simulink model "ConSys_A1"  (Simulink 8.3)
settings: Solver=ode3  StartTime=0.0  StopTime=Time(end)  FixedStep=Ts  RelTol=1e-3
values from neighbouring files (symbols this model uses):
  d = r*h    (= 1.6)    [StartUp_A1.m]
  d0 = d*h    (= 0.0032)    [StartUp_A1.m]
  h = 0.002    [StartUp_A1.m]
  Ka = diag([ 3  20  20  150  355  520])    [StartUp_A1.m]
  Kd = diag([ 3   5  25  100   15 1050])    [StartUp_A1.m]
  Ki = diag([35 555 810 7410 1850 5815])    [StartUp_A1.m]
  Kp = diag([55 180 350 1960  680 4450])    [StartUp_A1.m]
  r = 800    [StartUp_A1.m]
  TD = ss(Atd,Btd,Ctd,Dtd,Ts)    [StartUp_A1.m]
  Ts = 1/200    (= 0.005)    [StartUp_A1.m]
undefined symbols (not defined in the file or in its folder): DiscIntNeverNeededParam
undefined symbols (not defined in the file): ADAMS_cwd, ADAMS_exec, ADAMS_host, ADAMS_init, ADAMS_inputs, ADAMS_outputs, ADAMS_prefix, ADAMS_static, ADAMS_sysdir
libraries: cstblocks x6
(part 2 of 9)

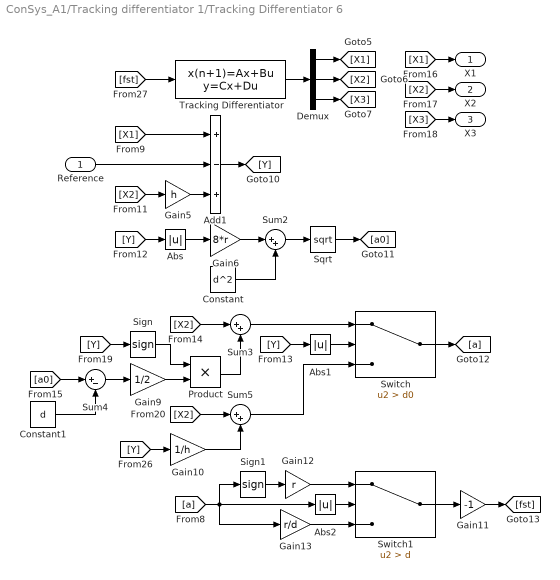
== system ConSys_A1/Tracking differentiator 1/Tracking Differentiator 6 ==
  Reference : Inport
  Abs : Abs
  Abs1 : Abs
  Abs2 : Abs
  Add1 : Sum  Inputs=+-+
  Constant : Constant  Value=d^2
  Constant1 : Constant  Value=d
  Demux : Demux  Outputs=3
  Gain10 : Gain  Gain=1/h
  Gain11 : Gain  Gain=-1
  Gain12 : Gain  Gain=r
  Gain13 : Gain  Gain=r/d
  Gain5 : Gain  Gain=h
  Gain6 : Gain  Gain=8*r
  Gain9 : Gain  Gain=1/2
  Product : Product
  Sign : Signum
  Sign1 : Signum
  Sqrt : Sqrt  SaturateOnIntegerOverflow=on
  Sum2 : Sum  Inputs=|++
  Sum3 : Sum  Inputs=|++
  Sum4 : Sum  Inputs=|+-
  Sum5 : Sum  Inputs=|++
  Switch : Switch  Criteria=u2 > Threshold  Threshold=d0
  Switch1 : Switch  Criteria=u2 > Threshold  Threshold=d
  Tracking Differentiator : DiscreteStateSpace  A=TD.a  B=TD.b  C=TD.c  D=TD.d  SampleTime=Ts
  X1 : Outport
  X2 : Outport  Port=2
  X3 : Outport  Port=3
  wires:
  Gain11/1 -> [fst]
  Abs2/1 -> Switch1/2
  [Y] -> Gain10/1
  Sum5/1 -> Switch/3
  Switch/1 -> [a]
  [Y] -> Sign/1
  Switch1/1 -> Gain11/1
  [a] -> Abs2/1, Sign1/1, Gain13/1
  Gain10/1 -> Sum5/2
  [fst] -> Tracking Differentiator/1
  [X2] -> Sum5/1
  Constant1/1 -> Sum4/2
  Sign/1 -> Product/1
  Product/1 -> Sum3/2
  [a0] -> Sum4/1
  Gain13/1 -> Switch1/3
  Sum4/1 -> Gain9/1
  [X2] -> Sum3/1
  Sum3/1 -> Switch/1
  [Y] -> Abs1/1
  Gain9/1 -> Product/2
  Sign1/1 -> Gain12/1
  Abs1/1 -> Switch/2
  Sum2/1 -> Sqrt/1
  Sqrt/1 -> [a0]
  Constant/1 -> Sum2/2
  Abs/1 -> Gain6/1
  Gain6/1 -> Sum2/1
  [Y] -> Abs/1
  Demux/2 -> [X2]
  Tracking Differentiator/1 -> Demux/1
  Demux/3 -> [X3]
  Demux/1 -> [X1]
  Add1/1 -> [Y]
  [X1] -> X1/1
  Reference/1 -> Add1/2
  [X2] -> Gain5/1
  [X2] -> X2/1
  Gain12/1 -> Switch1/1
  [X1] -> Add1/1
  Gain5/1 -> Add1/3
  [X3] -> X3/1

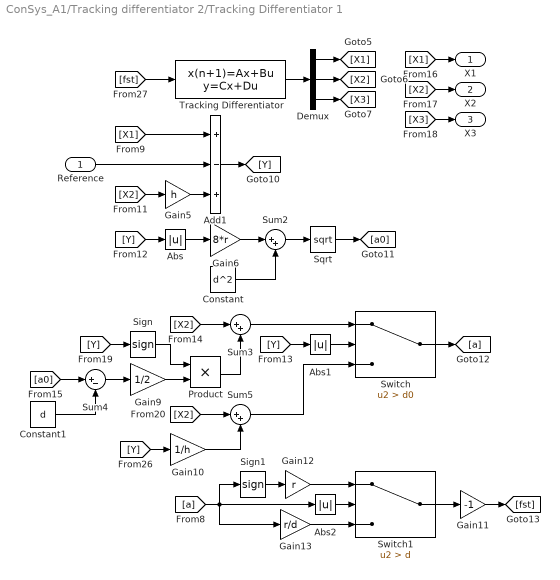
== system ConSys_A1/Tracking differentiator 2/Tracking Differentiator 1 ==
  Reference : Inport
  Abs : Abs
  Abs1 : Abs
  Abs2 : Abs
  Add1 : Sum  Inputs=+-+
  Constant : Constant  Value=d^2
  Constant1 : Constant  Value=d
  Demux : Demux  Outputs=3
  Gain10 : Gain  Gain=1/h
  Gain11 : Gain  Gain=-1
  Gain12 : Gain  Gain=r
  Gain13 : Gain  Gain=r/d
  Gain5 : Gain  Gain=h
  Gain6 : Gain  Gain=8*r
  Gain9 : Gain  Gain=1/2
  Product : Product
  Sign : Signum
  Sign1 : Signum
  Sqrt : Sqrt  SaturateOnIntegerOverflow=on
  Sum2 : Sum  Inputs=|++
  Sum3 : Sum  Inputs=|++
  Sum4 : Sum  Inputs=|+-
  Sum5 : Sum  Inputs=|++
  Switch : Switch  Criteria=u2 > Threshold  Threshold=d0
  Switch1 : Switch  Criteria=u2 > Threshold  Threshold=d
  Tracking Differentiator : DiscreteStateSpace  A=TD.a  B=TD.b  C=TD.c  D=TD.d  SampleTime=Ts
  X1 : Outport
  X2 : Outport  Port=2
  X3 : Outport  Port=3
  wires:
  Gain11/1 -> [fst]
  Abs2/1 -> Switch1/2
  [Y] -> Gain10/1
  Sum5/1 -> Switch/3
  Switch/1 -> [a]
  [Y] -> Sign/1
  Switch1/1 -> Gain11/1
  [a] -> Abs2/1, Sign1/1, Gain13/1
  Gain10/1 -> Sum5/2
  [fst] -> Tracking Differentiator/1
  [X2] -> Sum5/1
  Constant1/1 -> Sum4/2
  Sign/1 -> Product/1
  Product/1 -> Sum3/2
  [a0] -> Sum4/1
  Gain13/1 -> Switch1/3
  Sum4/1 -> Gain9/1
  [X2] -> Sum3/1
  Sum3/1 -> Switch/1
  [Y] -> Abs1/1
  Gain9/1 -> Product/2
  Sign1/1 -> Gain12/1
  Abs1/1 -> Switch/2
  Sum2/1 -> Sqrt/1
  Sqrt/1 -> [a0]
  Constant/1 -> Sum2/2
  Abs/1 -> Gain6/1
  Gain6/1 -> Sum2/1
  [Y] -> Abs/1
  Demux/2 -> [X2]
  Tracking Differentiator/1 -> Demux/1
  Demux/3 -> [X3]
  Demux/1 -> [X1]
  Add1/1 -> [Y]
  [X1] -> X1/1
  Reference/1 -> Add1/2
  [X2] -> Gain5/1
  [X2] -> X2/1
  Gain12/1 -> Switch1/1
  [X1] -> Add1/1
  Gain5/1 -> Add1/3
  [X3] -> X3/1

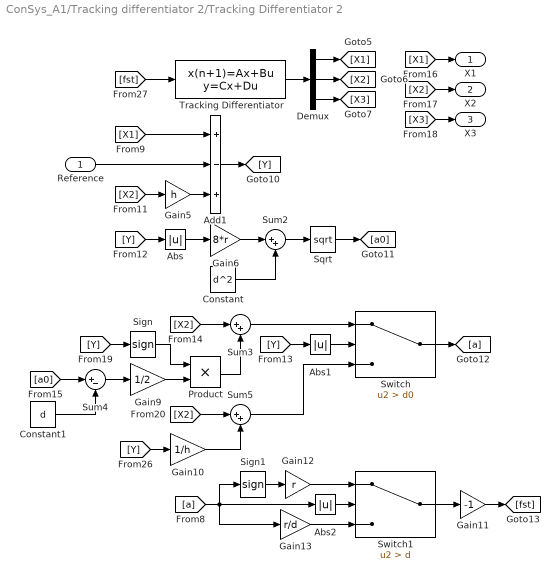
== system ConSys_A1/Tracking differentiator 2/Tracking Differentiator 2 ==
  Reference : Inport
  Abs : Abs
  Abs1 : Abs
  Abs2 : Abs
  Add1 : Sum  Inputs=+-+
  Constant : Constant  Value=d^2
  Constant1 : Constant  Value=d
  Demux : Demux  Outputs=3
  Gain10 : Gain  Gain=1/h
  Gain11 : Gain  Gain=-1
  Gain12 : Gain  Gain=r
  Gain13 : Gain  Gain=r/d
  Gain5 : Gain  Gain=h
  Gain6 : Gain  Gain=8*r
  Gain9 : Gain  Gain=1/2
  Product : Product
  Sign : Signum
  Sign1 : Signum
  Sqrt : Sqrt  SaturateOnIntegerOverflow=on
  Sum2 : Sum  Inputs=|++
  Sum3 : Sum  Inputs=|++
  Sum4 : Sum  Inputs=|+-
  Sum5 : Sum  Inputs=|++
  Switch : Switch  Criteria=u2 > Threshold  Threshold=d0
  Switch1 : Switch  Criteria=u2 > Threshold  Threshold=d
  Tracking Differentiator : DiscreteStateSpace  A=TD.a  B=TD.b  C=TD.c  D=TD.d  SampleTime=Ts
  X1 : Outport
  X2 : Outport  Port=2
  X3 : Outport  Port=3
  wires:
  [X3] -> X3/1
  Gain5/1 -> Add1/3
  [X1] -> Add1/1
  Gain12/1 -> Switch1/1
  [X2] -> X2/1
  [X2] -> Gain5/1
  Reference/1 -> Add1/2
  [X1] -> X1/1
  Add1/1 -> [Y]
  Demux/1 -> [X1]
  Demux/3 -> [X3]
  Tracking Differentiator/1 -> Demux/1
  Demux/2 -> [X2]
  [Y] -> Abs/1
  Gain6/1 -> Sum2/1
  Abs/1 -> Gain6/1
  Constant/1 -> Sum2/2
  Sqrt/1 -> [a0]
  Sum2/1 -> Sqrt/1
  Abs1/1 -> Switch/2
  Sign1/1 -> Gain12/1
  Gain9/1 -> Product/2
  [Y] -> Abs1/1
  Sum3/1 -> Switch/1
  [X2] -> Sum3/1
  Sum4/1 -> Gain9/1
  Gain13/1 -> Switch1/3
  [a0] -> Sum4/1
  Product/1 -> Sum3/2
  Sign/1 -> Product/1
  Constant1/1 -> Sum4/2
  [X2] -> Sum5/1
  [fst] -> Tracking Differentiator/1
  Gain10/1 -> Sum5/2
  [a] -> Gain13/1, Sign1/1, Abs2/1
  Switch1/1 -> Gain11/1
  [Y] -> Sign/1
  Switch/1 -> [a]
  Sum5/1 -> Switch/3
  [Y] -> Gain10/1
  Abs2/1 -> Switch1/2
  Gain11/1 -> [fst]

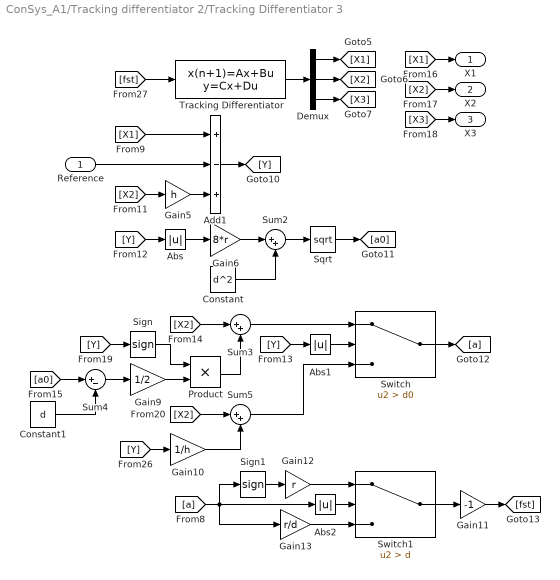
== system ConSys_A1/Tracking differentiator 2/Tracking Differentiator 3 ==
  Reference : Inport
  Abs : Abs
  Abs1 : Abs
  Abs2 : Abs
  Add1 : Sum  Inputs=+-+
  Constant : Constant  Value=d^2
  Constant1 : Constant  Value=d
  Demux : Demux  Outputs=3
  Gain10 : Gain  Gain=1/h
  Gain11 : Gain  Gain=-1
  Gain12 : Gain  Gain=r
  Gain13 : Gain  Gain=r/d
  Gain5 : Gain  Gain=h
  Gain6 : Gain  Gain=8*r
  Gain9 : Gain  Gain=1/2
  Product : Product
  Sign : Signum
  Sign1 : Signum
  Sqrt : Sqrt  SaturateOnIntegerOverflow=on
  Sum2 : Sum  Inputs=|++
  Sum3 : Sum  Inputs=|++
  Sum4 : Sum  Inputs=|+-
  Sum5 : Sum  Inputs=|++
  Switch : Switch  Criteria=u2 > Threshold  Threshold=d0
  Switch1 : Switch  Criteria=u2 > Threshold  Threshold=d
  Tracking Differentiator : DiscreteStateSpace  A=TD.a  B=TD.b  C=TD.c  D=TD.d  SampleTime=Ts
  X1 : Outport
  X2 : Outport  Port=2
  X3 : Outport  Port=3
  wires:
  Gain11/1 -> [fst]
  Abs2/1 -> Switch1/2
  [Y] -> Gain10/1
  Sum5/1 -> Switch/3
  Switch/1 -> [a]
  [Y] -> Sign/1
  Switch1/1 -> Gain11/1
  [a] -> Abs2/1, Sign1/1, Gain13/1
  Gain10/1 -> Sum5/2
  [fst] -> Tracking Differentiator/1
  [X2] -> Sum5/1
  Constant1/1 -> Sum4/2
  Sign/1 -> Product/1
  Product/1 -> Sum3/2
  [a0] -> Sum4/1
  Gain13/1 -> Switch1/3
  Sum4/1 -> Gain9/1
  [X2] -> Sum3/1
  Sum3/1 -> Switch/1
  [Y] -> Abs1/1
  Gain9/1 -> Product/2
  Sign1/1 -> Gain12/1
  Abs1/1 -> Switch/2
  Sum2/1 -> Sqrt/1
  Sqrt/1 -> [a0]
  Constant/1 -> Sum2/2
  Abs/1 -> Gain6/1
  Gain6/1 -> Sum2/1
  [Y] -> Abs/1
  Demux/2 -> [X2]
  Tracking Differentiator/1 -> Demux/1
  Demux/3 -> [X3]
  Demux/1 -> [X1]
  Add1/1 -> [Y]
  [X1] -> X1/1
  Reference/1 -> Add1/2
  [X2] -> Gain5/1
  [X2] -> X2/1
  Gain12/1 -> Switch1/1
  [X1] -> Add1/1
  Gain5/1 -> Add1/3
  [X3] -> X3/1

== system ConSys_A1/Tracking differentiator 2/Tracking Differentiator 4 ==
  Reference : Inport
  Abs : Abs
  Abs1 : Abs
  Abs2 : Abs
  Add1 : Sum  Inputs=+-+
  Constant : Constant  Value=d^2
  Constant1 : Constant  Value=d
  Demux : Demux  Outputs=3
  Gain10 : Gain  Gain=1/h
  Gain11 : Gain  Gain=-1
  Gain12 : Gain  Gain=r
  Gain13 : Gain  Gain=r/d
  Gain5 : Gain  Gain=h
  Gain6 : Gain  Gain=8*r
  Gain9 : Gain  Gain=1/2
  Product : Product
  Sign : Signum
  Sign1 : Signum
  Sqrt : Sqrt  SaturateOnIntegerOverflow=on
  Sum2 : Sum  Inputs=|++
  Sum3 : Sum  Inputs=|++
  Sum4 : Sum  Inputs=|+-
  Sum5 : Sum  Inputs=|++
  Switch : Switch  Criteria=u2 > Threshold  Threshold=d0
  Switch1 : Switch  Criteria=u2 > Threshold  Threshold=d
  Tracking Differentiator : DiscreteStateSpace  A=TD.a  B=TD.b  C=TD.c  D=TD.d  SampleTime=Ts
  X1 : Outport
  X2 : Outport  Port=2
  X3 : Outport  Port=3
  wires:
  [X3] -> X3/1
  Gain5/1 -> Add1/3
  [X1] -> Add1/1
  Gain12/1 -> Switch1/1
  [X2] -> X2/1
  [X2] -> Gain5/1
  Reference/1 -> Add1/2
  [X1] -> X1/1
  Add1/1 -> [Y]
  Demux/1 -> [X1]
  Demux/3 -> [X3]
  Tracking Differentiator/1 -> Demux/1
  Demux/2 -> [X2]
  [Y] -> Abs/1
  Gain6/1 -> Sum2/1
  Abs/1 -> Gain6/1
  Constant/1 -> Sum2/2
  Sqrt/1 -> [a0]
  Sum2/1 -> Sqrt/1
  Abs1/1 -> Switch/2
  Sign1/1 -> Gain12/1
  Gain9/1 -> Product/2
  [Y] -> Abs1/1
  Sum3/1 -> Switch/1
  [X2] -> Sum3/1
  Sum4/1 -> Gain9/1
  Gain13/1 -> Switch1/3
  [a0] -> Sum4/1
  Product/1 -> Sum3/2
  Sign/1 -> Product/1
  Constant1/1 -> Sum4/2
  [X2] -> Sum5/1
  [fst] -> Tracking Differentiator/1
  Gain10/1 -> Sum5/2
  [a] -> Gain13/1, Sign1/1, Abs2/1
  Switch1/1 -> Gain11/1
  [Y] -> Sign/1
  Switch/1 -> [a]
  Sum5/1 -> Switch/3
  [Y] -> Gain10/1
  Abs2/1 -> Switch1/2
  Gain11/1 -> [fst]

== system ConSys_A1/Tracking differentiator 2/Tracking Differentiator 5 ==
  Reference : Inport
  Abs : Abs
  Abs1 : Abs
  Abs2 : Abs
  Add1 : Sum  Inputs=+-+
  Constant : Constant  Value=d^2
  Constant1 : Constant  Value=d
  Demux : Demux  Outputs=3
  Gain10 : Gain  Gain=1/h
  Gain11 : Gain  Gain=-1
  Gain12 : Gain  Gain=r
  Gain13 : Gain  Gain=r/d
  Gain5 : Gain  Gain=h
  Gain6 : Gain  Gain=8*r
  Gain9 : Gain  Gain=1/2
  Product : Product
  Sign : Signum
  Sign1 : Signum
  Sqrt : Sqrt  SaturateOnIntegerOverflow=on
  Sum2 : Sum  Inputs=|++
  Sum3 : Sum  Inputs=|++
  Sum4 : Sum  Inputs=|+-
  Sum5 : Sum  Inputs=|++
  Switch : Switch  Criteria=u2 > Threshold  Threshold=d0
  Switch1 : Switch  Criteria=u2 > Threshold  Threshold=d
  Tracking Differentiator : DiscreteStateSpace  A=TD.a  B=TD.b  C=TD.c  D=TD.d  SampleTime=Ts
  X1 : Outport
  X2 : Outport  Port=2
  X3 : Outport  Port=3
  wires:
  Gain11/1 -> [fst]
  Abs2/1 -> Switch1/2
  [Y] -> Gain10/1
  Sum5/1 -> Switch/3
  Switch/1 -> [a]
  [Y] -> Sign/1
  Switch1/1 -> Gain11/1
  [a] -> Abs2/1, Sign1/1, Gain13/1
  Gain10/1 -> Sum5/2
  [fst] -> Tracking Differentiator/1
  [X2] -> Sum5/1
  Constant1/1 -> Sum4/2
  Sign/1 -> Product/1
  Product/1 -> Sum3/2
  [a0] -> Sum4/1
  Gain13/1 -> Switch1/3
  Sum4/1 -> Gain9/1
  [X2] -> Sum3/1
  Sum3/1 -> Switch/1
  [Y] -> Abs1/1
  Gain9/1 -> Product/2
  Sign1/1 -> Gain12/1
  Abs1/1 -> Switch/2
  Sum2/1 -> Sqrt/1
  Sqrt/1 -> [a0]
  Constant/1 -> Sum2/2
  Abs/1 -> Gain6/1
  Gain6/1 -> Sum2/1
  [Y] -> Abs/1
  Demux/2 -> [X2]
  Tracking Differentiator/1 -> Demux/1
  Demux/3 -> [X3]
  Demux/1 -> [X1]
  Add1/1 -> [Y]
  [X1] -> X1/1
  Reference/1 -> Add1/2
  [X2] -> Gain5/1
  [X2] -> X2/1
  Gain12/1 -> Switch1/1
  [X1] -> Add1/1
  Gain5/1 -> Add1/3
  [X3] -> X3/1

== system ConSys_A1/Tracking differentiator 2/Tracking Differentiator 6 ==
  Reference : Inport
  Abs : Abs
  Abs1 : Abs
  Abs2 : Abs
  Add1 : Sum  Inputs=+-+
  Constant : Constant  Value=d^2
  Constant1 : Constant  Value=d
  Demux : Demux  Outputs=3
  Gain10 : Gain  Gain=1/h
  Gain11 : Gain  Gain=-1
  Gain12 : Gain  Gain=r
  Gain13 : Gain  Gain=r/d
  Gain5 : Gain  Gain=h
  Gain6 : Gain  Gain=8*r
  Gain9 : Gain  Gain=1/2
  Product : Product
  Sign : Signum
  Sign1 : Signum
  Sqrt : Sqrt  SaturateOnIntegerOverflow=on
  Sum2 : Sum  Inputs=|++
  Sum3 : Sum  Inputs=|++
  Sum4 : Sum  Inputs=|+-
  Sum5 : Sum  Inputs=|++
  Switch : Switch  Criteria=u2 > Threshold  Threshold=d0
  Switch1 : Switch  Criteria=u2 > Threshold  Threshold=d
  Tracking Differentiator : DiscreteStateSpace  A=TD.a  B=TD.b  C=TD.c  D=TD.d  SampleTime=Ts
  X1 : Outport
  X2 : Outport  Port=2
  X3 : Outport  Port=3
  wires:
  [X3] -> X3/1
  Gain5/1 -> Add1/3
  [X1] -> Add1/1
  Gain12/1 -> Switch1/1
  [X2] -> X2/1
  [X2] -> Gain5/1
  Reference/1 -> Add1/2
  [X1] -> X1/1
  Add1/1 -> [Y]
  Demux/1 -> [X1]
  Demux/3 -> [X3]
  Tracking Differentiator/1 -> Demux/1
  Demux/2 -> [X2]
  [Y] -> Abs/1
  Gain6/1 -> Sum2/1
  Abs/1 -> Gain6/1
  Constant/1 -> Sum2/2
  Sqrt/1 -> [a0]
  Sum2/1 -> Sqrt/1
  Abs1/1 -> Switch/2
  Sign1/1 -> Gain12/1
  Gain9/1 -> Product/2
  [Y] -> Abs1/1
  Sum3/1 -> Switch/1
  [X2] -> Sum3/1
  Sum4/1 -> Gain9/1
  Gain13/1 -> Switch1/3
  [a0] -> Sum4/1
  Product/1 -> Sum3/2
  Sign/1 -> Product/1
  Constant1/1 -> Sum4/2
  [X2] -> Sum5/1
  [fst] -> Tracking Differentiator/1
  Gain10/1 -> Sum5/2
  [a] -> Gain13/1, Sign1/1, Abs2/1
  Switch1/1 -> Gain11/1
  [Y] -> Sign/1
  Switch/1 -> [a]
  Sum5/1 -> Switch/3
  [Y] -> Gain10/1
  Abs2/1 -> Switch1/2
  Gain11/1 -> [fst]

== matlab function A/MATLAB Function 2 ==
  data: q input double; M22 output double; M23 output double; M24 output double; M25 output double; M26 output double
function [M22,M23,M24,M25,M26] = M2(q)
%#codegen
Th1=q(1,1); Th2=q(2,1); Th3=q(3,1);
Th4=q(4,1); Th5=q(5,1); Th6=q(6,1);
M22=3.04e-8*sin(2.0*Th5) - 0.011534*cos(Th3) + 0.018628*cos(Th5) + 0.22909*sin(Th3) - 0.0000152*sin(Th5) + 0.01158*cos(Th4)^2 + 0.0066904*cos(Th5)^2 - 0.0066904*cos(Th4)^2*cos(Th5)^2 - 2.9736e-6*cos(Th4)^2*cos(Th6)^2 + 2.9736e-6*cos(Th5)^2*cos(Th6)^2 + 0.0004464*cos(Th3)*sin(Th4) + 0.017647*cos(Th5)*sin(Th3) + 0.0000874*cos(Th6)*sin(Th5) - 0.0000144*sin(Th3)*sin(Th5) + 0.0000144*cos(Th3)*cos(Th4)*cos(Th5) + 0.017647*cos(Th3)*cos(Th4)*sin(Th5) + 2.48e-8*cos(Th4)*cos(Th5)*sin(Th4) + 0.000019974*cos(Th5)*cos(Th6)*sin(Th5) - 2.9736e-6*cos(Th4)^2*cos(Th5)^2*cos(Th6)^2 + 0.0000828*cos(Th3)*sin(Th4)*sin(Th6) + 0.000078115*cos(Th4)*sin(Th4)*sin(Th5) + 0.0000828*cos(Th6)*sin(Th3)*sin(Th5) - 6.08e-8*cos(Th4)^2*cos(Th5)*sin(Th5) - 0.0000828*cos(Th3)*cos(Th4)*cos(Th5)*cos(Th6) + 0.000019974*cos(Th4)*sin(Th4)*sin(Th5)*sin(Th6) - 0.000019974*cos(Th4)^2*cos(Th5)*cos(Th6)*sin(Th5) + 5.9471e-6*cos(Th4)*cos(Th5)*cos(Th6)*sin(Th4)*sin(Th6) + 9.5038;
M23=3.04e-8*sin(2.0*Th5) - 0.0057672*cos(Th3) + 0.018628*cos(Th5) + 0.11454*sin(Th3) - 0.0000152*sin(Th5) + 0.01158*cos(Th4)^2 + 0.0066904*cos(Th5)^2 - 0.0066904*cos(Th4)^2*cos(Th5)^2 - 2.9736e-6*cos(Th4)^2*cos(Th6)^2 + 2.9736e-6*cos(Th5)^2*cos(Th6)^2 + 0.0002232*cos(Th3)*sin(Th4) + 0.0088236*cos(Th5)*sin(Th3) + 0.0000874*cos(Th6)*sin(Th5) - 7.2e-6*sin(Th3)*sin(Th5) + 7.2e-6*cos(Th3)*cos(Th4)*cos(Th5) + 0.0088236*cos(Th3)*cos(Th4)*sin(Th5) + 2.48e-8*cos(Th4)*cos(Th5)*sin(Th4) + 0.000019974*cos(Th5)*cos(Th6)*sin(Th5) - 2.9736e-6*cos(Th4)^2*cos(Th5)^2*cos(Th6)^2 + 0.0000414*cos(Th3)*sin(Th4)*sin(Th6) + 0.000078115*cos(Th4)*sin(Th4)*sin(Th5) + 0.0000414*cos(Th6)*sin(Th3)*sin(Th5) - 6.08e-8*cos(Th4)^2*cos(Th5)*sin(Th5) - 0.0000414*cos(Th3)*cos(Th4)*cos(Th5)*cos(Th6) + 0.000019974*cos(Th4)*sin(Th4)*sin(Th5)*sin(Th6) - 0.000019974*cos(Th4)^2*cos(Th5)*cos(Th6)*sin(Th5) + 5.9471e-6*cos(Th4)*cos(Th5)*cos(Th6)*sin(Th4)*sin(Th6) + 4.0591;
M24=0.0002356*cos(Th4) - 3.04e-8*sin(Th4) + 6.08e-8*cos(Th5)^2*sin(Th4) + 0.000039058*cos(Th4)*cos(Th5) + 0.0002232*cos(Th4)*sin(Th3) - 1.24e-8*cos(Th4)*sin(Th5) - 7.6e-6*cos(Th5)*sin(Th4) + 0.0000437*cos(Th4)*sin(Th6) - 9.9869e-6*cos(Th6)*sin(Th4) - 0.0093138*sin(Th4)*sin(Th5) + 9.9869e-6*cos(Th4)*cos(Th5)*sin(Th6) + 0.0000437*cos(Th5)*cos(Th6)*sin(Th4) - 7.2e-6*cos(Th5)*sin(Th3)*sin(Th4) + 0.0000414*cos(Th4)*sin(Th3)*sin(Th6) - 0.0066904*cos(Th5)*sin(Th4)*sin(Th5) - 0.0088236*sin(Th3)*sin(Th4)*sin(Th5) + 0.000019974*cos(Th5)^2*cos(Th6)*sin(Th4) + 0.0000414*cos(Th5)*cos(Th6)*sin(Th3)*sin(Th4) - 2.9736e-6*cos(Th4)*cos(Th6)*sin(Th5)*sin(Th6) - 2.9736e-6*cos(Th5)*cos(Th6)^2*sin(Th4)*sin(Th5);
M25=0.0075924*cos(Th4) - 2.9736e-6*cos(Th4)*cos(Th6)^2 + 7.2e-6*cos(Th3)*cos(Th5) + 0.0093138*cos(Th4)*cos(Th5) + 0.0088236*cos(Th3)*sin(Th5) - 7.6e-6*cos(Th4)*sin(Th5) + 1.24e-8*cos(Th5)*sin(Th4) + 0.000039058*sin(Th4)*sin(Th5) - 0.0000414*cos(Th3)*cos(Th5)*cos(Th6) + 0.0088236*cos(Th4)*cos(Th5)*sin(Th3) + 0.0000437*cos(Th4)*cos(Th6)*sin(Th5) - 7.2e-6*cos(Th4)*sin(Th3)*sin(Th5) + 9.9869e-6*sin(Th4)*sin(Th5)*sin(Th6) + 0.0000414*cos(Th4)*cos(Th6)*sin(Th3)*sin(Th5) + 2.9736e-6*cos(Th5)*cos(Th6)*sin(Th4)*sin(Th6);
M26=9.9869e-6*cos(Th4)*sin(Th6) + 0.0000437*cos(Th6)*sin(Th4) + 0.00011603*sin(Th4)*sin(Th5) + 0.0000437*cos(Th4)*cos(Th5)*sin(Th6) + 9.9869e-6*cos(Th5)*cos(Th6)*sin(Th4) + 0.0000414*cos(Th6)*sin(Th3)*sin(Th4) + 0.0000414*cos(Th3)*sin(Th5)*sin(Th6) + 0.0000414*cos(Th4)*cos(Th5)*sin(Th3)*sin(Th6);
end

== matlab function A/MATLAB Function 1 ==
  data: q input double; M11 output double; M12 output double; M13 output double; M14 output double; M15 output double; M16 output double
function [M11,M12,M13,M14,M15,M16] = M1(q)
%#codegen
Th1=q(1,1); Th2=q(2,1); Th3=q(3,1);
Th4=q(4,1); Th5=q(5,1); Th6=q(6,1);
M11=1.381*sin(Th2)^2 - 0.69402*sin(Th2) - 0.61644*cos(Th2)^2 - 0.034055*cos(Th2) + 0.011125*cos(Th2 + Th3)^2*cos(Th4)^2 + 0.01253*cos(Th2 + Th3)*sin(Th2 + Th3) + 0.015718*cos(Th2 + Th3)^2*sin(Th4)^2 + (0.00152*sin(Th5)*(sin(Th1)*sin(Th4) - 1.0*sin(Th2 + Th3)*cos(Th1)*cos(Th4)) - 0.00002*cos(Th5)*(sin(Th1)*sin(Th4) - 1.0*sin(Th2 + Th3)*cos(Th1)*cos(Th4)) - 0.07*cos(Th1) - 0.126*cos(Th2 + Th3)*cos(Th1) + 0.36*cos(Th1)*sin(Th2) + 0.00062*cos(Th4)*sin(Th1) + 0.00152*cos(Th2 + Th3)*cos(Th1)*cos(Th5) + 0.00002*cos(Th2 + Th3)*cos(Th1)*sin(Th5) + 0.00062*sin(Th2 + Th3)*cos(Th1)*sin(Th4) - 0.254*cos(Th1)*cos(Th2)*cos(Th3) + 0.254*cos(Th1)*sin(Th2)*sin(Th3))^2 + (0.00002*cos(Th5)*(cos(Th1)*sin(Th4) + sin(Th2 + Th3)*cos(Th4)*sin(Th1)) - 0.126*cos(Th2 + Th3)*sin(Th1) - 0.07*sin(Th1) - 0.00152*sin(Th5)*(cos(Th1)*sin(Th4) + sin(Th2 + Th3)*cos(Th4)*sin(Th1)) - 0.00062*cos(Th1)*cos(Th4) + 0.36*sin(Th1)*sin(Th2) + 0.00152*cos(Th2 + Th3)*cos(Th5)*sin(Th1) + 0.00002*cos(Th2 + Th3)*sin(Th1)*sin(Th5) + 0.00062*sin(Th2 + Th3)*sin(Th1)*sin(Th4) - 0.254*cos(Th2)*cos(Th3)*sin(Th1) + 0.254*sin(Th1)*sin(Th2)*sin(Th3))^2 + (sin(Th2 + Th3)*cos(Th5) + cos(Th2 + Th3)*cos(Th4)*sin(Th5))*(0.000489*sin(Th2 + Th3)*cos(Th5) - 0.00004*cos(Th2 + Th3)*sin(Th4) + 0.000489*cos(Th2 + Th3)*cos(Th4)*sin(Th5)) + (0.004898*sin(Th2 + Th3)*sin(Th5) - 0.004898*cos(Th2 + Th3)*cos(Th4)*cos(Th5))*(sin(Th2 + Th3)*sin(Th5) - 1.0*cos(Th2 + Th3)*cos(Th4)*cos(Th5)) + 18.0*(0.00867*cos(Th1) + 0.07*sin(Th1) - 0.36*sin(Th1)*sin(Th2) - 0.13649*cos(Th2)*cos(Th3)*sin(Th1) + 0.00089*cos(Th2)*sin(Th1)*sin(Th3) + 0.00089*cos(Th3)*sin(Th1)*sin(Th2) + 0.13649*sin(Th1)*sin(Th2)*sin(Th3))^2 + 6.5*(0.07*cos(Th1) + 0.08523*cos(Th2 + Th3)*cos(Th1) - 0.36*cos(Th1)*sin(Th2) + 0.254*cos(Th1)*cos(Th2)*cos(Th3) - 0.254*cos(Th1)*sin(Th2)*sin(Th3))^2 + (sin(Th6)*(sin(Th2 + Th3)*sin(Th5) - 1.0*cos(Th2 + Th3)*cos(Th4)*cos(Th5)) - 1.0*cos(Th2 + Th3)*cos(Th6)*sin(Th4))*(0.00104*sin(Th6)*(sin(Th2 + Th3)*sin(Th5) - 1.0*cos(Th2 + Th3)*cos(Th4)*cos(Th5)) - 0.00104*cos(Th2 + Th3)*cos(Th6)*sin(Th4)) + 18.0*(0.07*cos(Th1) - 0.00867*sin(Th1) - 0.36*cos(Th1)*sin(Th2) - 0.13649*cos(Th1)*cos(Th2)*cos(Th3) + 0.00089*cos(Th1)*cos(Th2)*sin(Th3) + 0.00089*cos(Th1)*cos(Th3)*sin(Th2) + 0.13649*cos(Th1)*sin(Th2)*sin(Th3))^2 + 2.7583*cos(Th2 + Th3)^2 + 0.019393*sin(Th2 + Th3)^2 - 1.0*(sin(Th2 + Th3)*cos(Th5) + cos(Th2 + Th3)*cos(Th4)*sin(Th5))*(4.0e-6*cos(Th6)*(sin(Th2 + Th3)*sin(Th5) - 1.0*cos(Th2 + Th3)*cos(Th4)*cos(Th5)) - 0.000116*sin(Th2 + Th3)*cos(Th5) - 0.000116*cos(Th2 + Th3)*cos(Th4)*sin(Th5) + 4.0e-6*cos(Th2 + Th3)*sin(Th4)*sin(Th6)) + (cos(Th6)*(sin(Th2 + Th3)*sin(Th5) - 1.0*cos(Th2 + Th3)*cos(Th4)*cos(Th5)) + cos(Th2 + Th3)*sin(Th4)*sin(Th6))*(0.001043*cos(Th6)*(sin(Th2 + Th3)*sin(Th5) - 1.0*cos(Th2 + Th3)*cos(Th4)*cos(Th5)) - 4.0e-6*sin(Th2 + Th3)*cos(Th5) - 4.0e-6*cos(Th2 + Th3)*cos(Th4)*sin(Th5) + 0.001043*cos(Th2 + Th3)*sin(Th4)*sin(Th6)) + 0.18719*cos(Th2)*sin(Th2) + 0.5*(0.07*sin(Th1) + 0.00023*sin(Th6)*(cos(Th1)*cos(Th4) - 1.0*sin(Th2 + Th3)*sin(Th1)*sin(Th4)) + 0.00023*cos(Th6)*(cos(Th5)*(cos(Th1)*sin(Th4) + sin(Th2 + Th3)*cos(Th4)*sin(Th1)) + cos(Th2 + Th3)*sin(Th1)*sin(Th5)) + 0.126*cos(Th2 + Th3)*sin(Th1) - 0.05206*sin(Th5)*(cos(Th1)*sin(Th4) + sin(Th2 + Th3)*cos(Th4)*sin(Th1)) - 0.36*sin(Th1)*sin(Th2) + 0.05206*cos(Th2 + Th3)*cos(Th5)*sin(Th1) + 0.254*cos(Th2)*cos(Th3)*sin(Th1) - 0.254*sin(Th1)*sin(Th2)*sin(Th3))^2 + 0.5*(0.07*cos(Th1) + 0.05206*sin(Th5)*(sin(Th1)*sin(Th4) - 1.0*sin(Th2 + Th3)*cos(Th1)*cos(Th4)) + 0.126*cos(Th2 + Th3)*cos(Th1) - 0.00023*sin(Th6)*(cos(Th4)*sin(Th1) + sin(Th2 + Th3)*cos(Th1)*sin(Th4)) - 0.36*cos(Th1)*sin(Th2) - 0.00023*cos(Th6)*(cos(Th5)*(sin(Th1)*sin(Th4) - 1.0*sin(Th2 + Th3)*cos(Th1)*cos(Th4)) - 1.0*cos(Th2 + Th3)*cos(Th1)*sin(Th5)) + 0.05206*cos(Th2 + Th3)*cos(Th1)*cos(Th5) + 0.254*cos(Th1)*cos(Th2)*cos(Th3) - 0.254*cos(Th1)*sin(Th2)*sin(Th3))^2 + 6.5*(0.07*sin(Th1) + 0.08523*cos(Th2 + Th3)*sin(Th1) - 0.36*sin(Th1)*sin(Th2) + 0.254*cos(Th2)*cos(Th3)*sin(Th1) - 0.254*sin(Th1)*sin(Th2)*sin(Th3))^2 - 1.0*cos(Th2 + Th3)*sin(Th4)*(0.00004*sin(Th2 + Th3)*cos(Th5) - 0.005192*cos(Th2 + Th3)*sin(Th4) + 0.00004*cos(Th2 + Th3)*cos(Th4)*sin(Th5)) + 2.2957;
M12=0.00015211*cos(Th2 + Th3) + 0.039618*sin(Th2 + Th3) - 0.71642*cos(Th2) + 0.0017066*sin(Th2) + (0.00062*cos(Th4) - 0.00002*cos(Th5)*sin(Th4) + 0.00152*sin(Th4)*sin(Th5))*(0.126*sin(Th2 + Th3) + 0.36*cos(Th2) + 0.00062*cos(Th2 + Th3)*sin(Th4) - 0.00152*sin(Th2 + Th3)*cos(Th5) - 0.00002*sin(Th2 + Th3)*sin(Th5) + 0.254*cos(Th2)*sin(Th3) + 0.254*cos(Th3)*sin(Th2) + 0.00002*cos(Th2 + Th3)*cos(Th4)*cos(Th5) - 0.00152*cos(Th2 + Th3)*cos(Th4)*sin(Th5)) - 0.00004*cos(Th2 + Th3)*sin(Th5) + (0.000115*cos(Th4)*sin(Th6) - 0.02603*sin(Th4)*sin(Th5) + 0.000115*cos(Th5)*cos(Th6)*sin(Th4))*(0.126*sin(Th2 + Th3) + 0.36*cos(Th2) + 0.05206*sin(Th2 + Th3)*cos(Th5) + 0.254*cos(Th2)*sin(Th3) + 0.254*cos(Th3)*sin(Th2) + 0.05206*cos(Th2 + Th3)*cos(Th4)*sin(Th5) + 0.00023*cos(Th2 + Th3)*sin(Th4)*sin(Th6) + 0.00023*sin(Th2 + Th3)*cos(Th6)*sin(Th5) - 0.00023*cos(Th2 + Th3)*cos(Th4)*cos(Th5)*cos(Th6)) - 0.010223*cos(Th2 + Th3)*cos(Th4)*sin(Th4) + 0.00004*sin(Th2 + Th3)*cos(Th4)*cos(Th5) - 4.0e-6*sin(Th2 + Th3)*cos(Th6)*sin(Th4) - 4.0e-6*cos(Th2 + Th3)*sin(Th5)*sin(Th6) + 0.00008*cos(Th2 + Th3)*cos(Th4)^2*sin(Th5) - 3.0e-6*cos(Th2 + Th3)*cos(Th5)*cos(Th6)*sin(Th6) + 4.0e-6*sin(Th2 + Th3)*cos(Th4)*cos(Th5)*sin(Th6) - 0.005333*sin(Th2 + Th3)*cos(Th5)*sin(Th4)*sin(Th5) + 0.005333*cos(Th2 + Th3)*cos(Th4)*cos(Th5)^2*sin(Th4) + 3.0e-6*cos(Th2 + Th3)*cos(Th4)*cos(Th6)^2*sin(Th4) + 8.0e-6*cos(Th2 + Th3)*cos(Th4)^2*sin(Th5)*sin(Th6) + 8.0e-6*sin(Th2 + Th3)*cos(Th5)^2*cos(Th6)*sin(Th4) + 6.0e-6*cos(Th2 + Th3)*cos(Th4)^2*cos(Th5)*cos(Th6)*sin(Th6) - 3.0e-6*sin(Th2 + Th3)*cos(Th5)*cos(Th6)^2*sin(Th4)*sin(Th5) + 3.0e-6*cos(Th2 + Th3)*cos(Th4)*cos(Th5)^2*cos(Th6)^2*sin(Th4) - 3.0e-6*sin(Th2 + Th3)*cos(Th4)*cos(Th6)*sin(Th5)*sin(Th6) + 8.0e-6*cos(Th2 + Th3)*cos(Th4)*cos(Th5)*cos(Th6)*sin(Th4)*sin(Th5);
M13=0.00015211*cos(Th2 + Th3) + 0.039618*sin(Th2 + Th3) + (0.000115*cos(Th4)*sin(Th6) - 0.02603*sin(Th4)*sin(Th5) + 0.000115*cos(Th5)*cos(Th6)*sin(Th4))*(0.126*sin(Th2 + Th3) + 0.05206*sin(Th2 + Th3)*cos(Th5) + 0.254*cos(Th2)*sin(Th3) + 0.254*cos(Th3)*sin(Th2) + 0.05206*cos(Th2 + Th3)*cos(Th4)*sin(Th5) + 0.00023*cos(Th2 + Th3)*sin(Th4)*sin(Th6) + 0.00023*sin(Th2 + Th3)*cos(Th6)*sin(Th5) - 0.00023*cos(Th2 + Th3)*cos(Th4)*cos(Th5)*cos(Th6)) - 0.00004*cos(Th2 + Th3)*sin(Th5) + (0.00062*cos(Th4) - 0.00002*cos(Th5)*sin(Th4) + 0.00152*sin(Th4)*sin(Th5))*(0.126*sin(Th2 + Th3) + 0.00062*cos(Th2 + Th3)*sin(Th4) - 0.00152*sin(Th2 + Th3)*cos(Th5) - 0.00002*sin(Th2 + Th3)*sin(Th5) + 0.254*cos(Th2)*sin(Th3) + 0.254*cos(Th3)*sin(Th2) + 0.00002*cos(Th2 + Th3)*cos(Th4)*cos(Th5) - 0.00152*cos(Th2 + Th3)*cos(Th4)*sin(Th5)) - 0.010223*cos(Th2 + Th3)*cos(Th4)*sin(Th4) + 0.00004*sin(Th2 + Th3)*cos(Th4)*cos(Th5) - 4.0e-6*sin(Th2 + Th3)*cos(Th6)*sin(Th4) - 4.0e-6*cos(Th2 + Th3)*sin(Th5)*sin(Th6) + 0.00008*cos(Th2 + Th3)*cos(Th4)^2*sin(Th5) - 3.0e-6*cos(Th2 + Th3)*cos(Th5)*cos(Th6)*sin(Th6) + 4.0e-6*sin(Th2 + Th3)*cos(Th4)*cos(Th5)*sin(Th6) - 0.005333*sin(Th2 + Th3)*cos(Th5)*sin(Th4)*sin(Th5) + 0.005333*cos(Th2 + Th3)*cos(Th4)*cos(Th5)^2*sin(Th4) + 3.0e-6*cos(Th2 + Th3)*cos(Th4)*cos(Th6)^2*sin(Th4) + 8.0e-6*cos(Th2 + Th3)*cos(Th4)^2*sin(Th5)*sin(Th6) + 8.0e-6*sin(Th2 + Th3)*cos(Th5)^2*cos(Th6)*sin(Th4) + 6.0e-6*cos(Th2 + Th3)*cos(Th4)^2*cos(Th5)*cos(Th6)*sin(Th6) - 3.0e-6*sin(Th2 + Th3)*cos(Th5)*cos(Th6)^2*sin(Th4)*sin(Th5) + 3.0e-6*cos(Th2 + Th3)*cos(Th4)*cos(Th5)^2*cos(Th6)^2*sin(Th4) - 3.0e-6*sin(Th2 + Th3)*cos(Th4)*cos(Th6)*sin(Th5)*sin(Th6) + 8.0e-6*cos(Th2 + Th3)*cos(Th4)*cos(Th5)*cos(Th6)*sin(Th4)*sin(Th5);
M14=0.012239*cos(Th2)*sin(Th3) - 1.4e-6*cos(Th4)*cos(Th5) - 0.0000434*sin(Th4) + 0.012239*cos(Th3)*sin(Th2) - 0.0017157*cos(Th4)*sin(Th5) + 0.0002232*sin(Th2)*sin(Th4) - 8.05e-6*sin(Th4)*sin(Th6) - 3.04e-8*cos(Th2)*cos(Th3)*cos(Th4) + 8.05e-6*cos(Th4)*cos(Th5)*cos(Th6) - 0.0002356*cos(Th2)*cos(Th3)*sin(Th4) + 7.2e-6*cos(Th4)*cos(Th5)*sin(Th2) + 3.04e-8*cos(Th4)*sin(Th2)*sin(Th3) + 0.0088236*cos(Th4)*sin(Th2)*sin(Th5) + 0.0002356*sin(Th2)*sin(Th3)*sin(Th4) + 0.0000414*sin(Th2)*sin(Th4)*sin(Th6) - 0.0066904*cos(Th2)*cos(Th5)^2*sin(Th3) - 0.0066904*cos(Th3)*cos(Th5)^2*sin(Th2) + 2.9736e-6*cos(Th2)*cos(Th6)^2*sin(Th3) + 2.9736e-6*cos(Th3)*cos(Th6)^2*sin(Th2) - 2.9736e-6*cos(Th2)*cos(Th5)^2*cos(Th6)^2*sin(Th3) - 2.9736e-6*cos(Th3)*cos(Th5)^2*cos(Th6)^2*sin(Th2) - 7.6e-6*cos(Th2)*cos(Th3)*cos(Th4)*cos(Th5) - 9.9869e-6*cos(Th2)*cos(Th3)*cos(Th4)*cos(Th6) - 0.0093138*cos(Th2)*cos(Th3)*cos(Th4)*sin(Th5) - 0.000039058*cos(Th2)*cos(Th3)*cos(Th5)*sin(Th4) - 0.0000414*cos(Th4)*cos(Th5)*cos(Th6)*sin(Th2) + 1.24e-8*cos(Th2)*cos(Th3)*sin(Th4)*sin(Th5) + 7.6e-6*cos(Th4)*cos(Th5)*sin(Th2)*sin(Th3) - 0.0000437*cos(Th2)*cos(Th3)*sin(Th4)*sin(Th6) - 6.08e-8*cos(Th2)*cos(Th5)*sin(Th3)*sin(Th5) - 6.08e-8*cos(Th3)*cos(Th5)*sin(Th2)*sin(Th5) + 9.9869e-6*cos(Th4)*cos(Th6)*sin(Th2)*sin(Th3) + 0.0093138*cos(Th4)*sin(Th2)*sin(Th3)*sin(Th5) + 0.000039058*cos(Th5)*sin(Th2)*sin(Th3)*sin(Th4) - 1.24e-8*sin(Th2)*sin(Th3)*sin(Th4)*sin(Th5) + 0.0000437*sin(Th2)*sin(Th3)*sin(Th4)*sin(Th6) + 6.08e-8*cos(Th2)*cos(Th3)*cos(Th4)*cos(Th5)^2 - 6.08e-8*cos(Th4)*cos(Th5)^2*sin(Th2)*sin(Th3) - 0.0066904*cos(Th2)*cos(Th3)*cos(Th4)*cos(Th5)*sin(Th5) - 9.9869e-6*cos(Th2)*cos(Th3)*cos(Th5)*sin(Th4)*sin(Th6) - 0.0000437*cos(Th4)*cos(Th5)*cos(Th6)*sin(Th2)*sin(Th3) - 0.000019974*cos(Th2)*cos(Th5)*cos(Th6)*sin(Th3)*sin(Th5) - 0.000019974*cos(Th3)*cos(Th5)*cos(Th6)*sin(Th2)*sin(Th5) + 0.0066904*cos(Th4)*cos(Th5)*sin(Th2)*sin(Th3)*sin(Th5) + 9.9869e-6*cos(Th5)*sin(Th2)*sin(Th3)*sin(Th4)*sin(Th6) + 0.000019974*cos(Th2)*cos(Th3)*cos(Th4)*cos(Th5)^2*cos(Th6) - 0.000019974*cos(Th4)*cos(Th5)^2*cos(Th6)*sin(Th2)*sin(Th3) + 0.0000437*cos(Th2)*cos(Th3)*cos(Th4)*cos(Th5)*cos(Th6) - 2.9736e-6*cos(Th2)*cos(Th3)*cos(Th4)*cos(Th5)*cos(Th6)^2*sin(Th5) + 2.9736e-6*cos(Th4)*cos(Th5)*cos(Th6)^2*sin(Th2)*sin(Th3)*sin(Th5) + 2.9736e-6*cos(Th2)*cos(Th3)*cos(Th6)*sin(Th4)*sin(Th5)*sin(Th6) - 2.9736e-6*cos(Th6)*sin(Th2)*sin(Th3)*sin(Th4)*sin(Th5)*sin(Th6);
M15=1.4e-6*sin(Th4)*sin(Th5) - 0.0017157*cos(Th5)*sin(Th4) - 0.0075924*cos(Th2)*cos(Th3)*sin(Th4) + 0.000039058*cos(Th2)*cos(Th5)*sin(Th3) + 0.000039058*cos(Th3)*cos(Th5)*sin(Th2) - 1.24e-8*cos(Th2)*sin(Th3)*sin(Th5) - 1.24e-8*cos(Th3)*sin(Th2)*sin(Th5) + 0.0088236*cos(Th5)*sin(Th2)*sin(Th4) - 8.05e-6*cos(Th6)*sin(Th4)*sin(Th5) + 0.0075924*sin(Th2)*sin(Th3)*sin(Th4) - 7.2e-6*sin(Th2)*sin(Th4)*sin(Th5) + 1.24e-8*cos(Th2)*cos(Th3)*cos(Th4)*cos(Th5) + 0.000039058*cos(Th2)*cos(Th3)*cos(Th4)*sin(Th5) - 0.0093138*cos(Th2)*cos(Th3)*cos(Th5)*sin(Th4) + 7.6e-6*cos(Th2)*cos(Th3)*sin(Th4)*sin(Th5) - 1.24e-8*cos(Th4)*cos(Th5)*sin(Th2)*sin(Th3) + 9.9869e-6*cos(Th2)*cos(Th5)*sin(Th3)*sin(Th6) + 9.9869e-6*cos(Th3)*cos(Th5)*sin(Th2)*sin(Th6) - 0.000039058*cos(Th4)*sin(Th2)*sin(Th3)*sin(Th5) + 0.0093138*cos(Th5)*sin(Th2)*sin(Th3)*sin(Th4) + 0.0000414*cos(Th6)*sin(Th2)*sin(Th4)*sin(Th5) - 7.6e-6*sin(Th2)*sin(Th3)*sin(Th4)*sin(Th5) + 2.9736e-6*cos(Th2)*cos(Th3)*cos(Th6)^2*sin(Th4) - 2.9736e-6*cos(Th6)^2*sin(Th2)*sin(Th3)*sin(Th4) + 9.9869e-6*cos(Th2)*cos(Th3)*cos(Th4)*sin(Th5)*sin(Th6) - 0.0000437*cos(Th2)*cos(Th3)*cos(Th6)*sin(Th4)*sin(Th5) - 2.9736e-6*cos(Th2)*cos(Th6)*sin(Th3)*sin(Th5)*sin(Th6) - 2.9736e-6*cos(Th3)*cos(Th6)*sin(Th2)*sin(Th5)*sin(Th6) - 9.9869e-6*cos(Th4)*sin(Th2)*sin(Th3)*sin(Th5)*sin(Th6) + 0.0000437*cos(Th6)*sin(Th2)*sin(Th3)*sin(Th4)*sin(Th5) + 2.9736e-6*cos(Th2)*cos(Th3)*cos(Th4)*cos(Th5)*cos(Th6)*sin(Th6) - 2.9736e-6*cos(Th4)*cos(Th5)*cos(Th6)*sin(Th2)*sin(Th3)*sin(Th6);
M16=8.05e-6*cos(Th4)*cos(Th6) + 0.00011603*cos(Th2)*cos(Th5)*sin(Th3) + 0.00011603*cos(Th3)*cos(Th5)*sin(Th2) - 0.0000414*cos(Th4)*cos(Th6)*sin(Th2) - 8.05e-6*cos(Th5)*sin(Th4)*sin(Th6) + 0.0000437*cos(Th2)*cos(Th3)*cos(Th4)*cos(Th6) + 0.00011603*cos(Th2)*cos(Th3)*cos(Th4)*sin(Th5) - 9.9869e-6*cos(Th2)*cos(Th3)*sin(Th4)*sin(Th6) - 0.0000437*cos(Th4)*cos(Th6)*sin(Th2)*sin(Th3) - 9.9869e-6*cos(Th2)*cos(Th6)*sin(Th3)*sin(Th5) - 9.9869e-6*cos(Th3)*cos(Th6)*sin(Th2)*sin(Th5) - 0.00011603*cos(Th4)*sin(Th2)*sin(Th3)*sin(Th5) + 0.0000414*cos(Th5)*sin(Th2)*sin(Th4)*sin(Th6) + 9.9869e-6*sin(Th2)*sin(Th3)*sin(Th4)*sin(Th6) - 0.0000437*cos(Th2)*cos(Th3)*cos(Th5)*sin(Th4)*sin(Th6) - 9.9869e-6*cos(Th4)*cos(Th5)*cos(Th6)*sin(Th2)*sin(Th3) + 0.0000437*cos(Th5)*sin(Th2)*sin(Th3)*sin(Th4)*sin(Th6) + 9.9869e-6*cos(Th2)*cos(Th3)*cos(Th4)*cos(Th5)*cos(Th6);
% M61=M16; M31=M13; M41=M14; M51=M15; M21=M12;
end

== matlab function A/MATLAB Function 3 ==
  data: q input double; M33 output double; M34 output double; M35 output double; M36 output double
function [M33,M34,M35,M36] = M3(q)
%#codegen
Th1=q(1,1); Th2=q(2,1); Th3=q(3,1);
Th4=q(4,1); Th5=q(5,1); Th6=q(6,1);
M33=3.04e-8*sin(2.0*Th5) + 0.018628*cos(Th5) - 0.0000152*sin(Th5) + 0.01158*cos(Th4)^2 + 0.0066904*cos(Th5)^2 - 0.0066904*cos(Th4)^2*cos(Th5)^2 - 2.9736e-6*cos(Th4)^2*cos(Th6)^2 + 2.9736e-6*cos(Th5)^2*cos(Th6)^2 + 0.0000874*cos(Th6)*sin(Th5) + 2.48e-8*cos(Th4)*cos(Th5)*sin(Th4) + 0.000019974*cos(Th5)*cos(Th6)*sin(Th5) - 2.9736e-6*cos(Th4)^2*cos(Th5)^2*cos(Th6)^2 + 0.000078115*cos(Th4)*sin(Th4)*sin(Th5) - 6.08e-8*cos(Th4)^2*cos(Th5)*sin(Th5) + 0.000019974*cos(Th4)*sin(Th4)*sin(Th5)*sin(Th6) - 0.000019974*cos(Th4)^2*cos(Th5)*cos(Th6)*sin(Th5) + 5.9471e-6*cos(Th4)*cos(Th5)*cos(Th6)*sin(Th4)*sin(Th6) + 4.0591;
M34=0.0002356*cos(Th4) - 3.04e-8*sin(Th4) + 6.08e-8*cos(Th5)^2*sin(Th4) + 0.000039058*cos(Th4)*cos(Th5) - 1.24e-8*cos(Th4)*sin(Th5) - 7.6e-6*cos(Th5)*sin(Th4) + 0.0000437*cos(Th4)*sin(Th6) - 9.9869e-6*cos(Th6)*sin(Th4) - 0.0093138*sin(Th4)*sin(Th5) + 9.9869e-6*cos(Th4)*cos(Th5)*sin(Th6) + 0.0000437*cos(Th5)*cos(Th6)*sin(Th4) - 0.0066904*cos(Th5)*sin(Th4)*sin(Th5) + 0.000019974*cos(Th5)^2*cos(Th6)*sin(Th4) - 2.9736e-6*cos(Th4)*cos(Th6)*sin(Th5)*sin(Th6) - 2.9736e-6*cos(Th5)*cos(Th6)^2*sin(Th4)*sin(Th5);
M35=0.0075924*cos(Th4) - 2.9736e-6*cos(Th4)*cos(Th6)^2 + 0.0093138*cos(Th4)*cos(Th5) - 7.6e-6*cos(Th4)*sin(Th5) + 1.24e-8*cos(Th5)*sin(Th4) + 0.000039058*sin(Th4)*sin(Th5) + 0.0000437*cos(Th4)*cos(Th6)*sin(Th5) + 9.9869e-6*sin(Th4)*sin(Th5)*sin(Th6) + 2.9736e-6*cos(Th5)*cos(Th6)*sin(Th4)*sin(Th6);
M36=9.9869e-6*cos(Th4)*sin(Th6) + 0.0000437*cos(Th6)*sin(Th4) + 0.00011603*sin(Th4)*sin(Th5) + 0.0000437*cos(Th4)*cos(Th5)*sin(Th6) + 9.9869e-6*cos(Th5)*cos(Th6)*sin(Th4);
% M61=M16; M31=M13; M41=M14; M51=M15; M21=M12;
end

== matlab function A/MATLAB Function 4 ==
  data: q input double; M44 output double; M45 output double; M46 output double
function [M44,M45,M46] = M4(q)
%#codegen
Th1=q(1,1); Th2=q(2,1); Th3=q(3,1);
Th4=q(4,1); Th5=q(5,1); Th6=q(6,1);
M44=(0.00062*cos(Th1)*sin(Th4) + 0.00062*sin(Th2 + Th3)*cos(Th4)*sin(Th1) + 0.00002*cos(Th1)*cos(Th4)*cos(Th5) - 0.00152*cos(Th1)*cos(Th4)*sin(Th5) - 0.00002*sin(Th2 + Th3)*cos(Th5)*sin(Th1)*sin(Th4) + 0.00152*sin(Th2 + Th3)*sin(Th1)*sin(Th4)*sin(Th5))^2 - 0.005333*cos(Th5)^2 + 3.0e-6*cos(Th6)^2 + cos(Th2 + Th3)^2*(0.00062*cos(Th4) - 0.00002*cos(Th5)*sin(Th4) + 0.00152*sin(Th4)*sin(Th5))^2 + (0.00062*sin(Th1)*sin(Th4) - 0.00062*sin(Th2 + Th3)*cos(Th1)*cos(Th4) + 0.00002*cos(Th4)*cos(Th5)*sin(Th1) - 0.00152*cos(Th4)*sin(Th1)*sin(Th5) + 0.00002*sin(Th2 + Th3)*cos(Th1)*cos(Th5)*sin(Th4) - 0.00152*sin(Th2 + Th3)*cos(Th1)*sin(Th4)*sin(Th5))^2 + 0.5*(0.05206*cos(Th4)*sin(Th1)*sin(Th5) + 0.00023*sin(Th1)*sin(Th4)*sin(Th6) - 0.00023*sin(Th2 + Th3)*cos(Th1)*cos(Th4)*sin(Th6) + 0.05206*sin(Th2 + Th3)*cos(Th1)*sin(Th4)*sin(Th5) - 0.00023*cos(Th4)*cos(Th5)*cos(Th6)*sin(Th1) - 0.00023*sin(Th2 + Th3)*cos(Th1)*cos(Th5)*cos(Th6)*sin(Th4))^2 + 0.5*(0.05206*cos(Th1)*cos(Th4)*sin(Th5) + 0.00023*cos(Th1)*sin(Th4)*sin(Th6) + 0.00023*sin(Th2 + Th3)*cos(Th4)*sin(Th1)*sin(Th6) - 0.05206*sin(Th2 + Th3)*sin(Th1)*sin(Th4)*sin(Th5) - 0.00023*cos(Th1)*cos(Th4)*cos(Th5)*cos(Th6) + 0.00023*sin(Th2 + Th3)*cos(Th5)*cos(Th6)*sin(Th1)*sin(Th4))^2 - 3.0e-6*cos(Th5)^2*cos(Th6)^2 + 0.5*cos(Th2 + Th3)^2*(0.00023*cos(Th4)*sin(Th6) - 0.05206*sin(Th4)*sin(Th5) + 0.00023*cos(Th5)*cos(Th6)*sin(Th4))^2 - 8.0e-6*cos(Th5)*cos(Th6)*sin(Th5) + 0.010881;
M45=0.000039058*cos(Th5) - 1.24e-8*sin(Th5) + 9.9869e-6*cos(Th5)*sin(Th6) - 2.9736e-6*cos(Th6)*sin(Th5)*sin(Th6);
M46=(0.5*(sin(Th2 + Th3)*cos(Th5) + cos(Th2 + Th3)*cos(Th4)*sin(Th5))*(0.01294*sin(Th5)*(sin(Th1)*sin(Th4) - 1.0*sin(Th2 + Th3)*cos(Th1)*cos(Th4)) + 0.00023*sin(Th6)*(cos(Th4)*sin(Th1) + sin(Th2 + Th3)*cos(Th1)*sin(Th4)) + 0.00023*cos(Th6)*(cos(Th5)*(sin(Th1)*sin(Th4) - 1.0*sin(Th2 + Th3)*cos(Th1)*cos(Th4)) - 1.0*cos(Th2 + Th3)*cos(Th1)*sin(Th5)) + 0.01294*cos(Th2 + Th3)*cos(Th1)*cos(Th5)) + 0.5*(sin(Th5)*(sin(Th1)*sin(Th4) - 1.0*sin(Th2 + Th3)*cos(Th1)*cos(Th4)) + cos(Th2 + Th3)*cos(Th1)*cos(Th5))*(0.00023*cos(Th6)*(sin(Th2 + Th3)*sin(Th5) - 1.0*cos(Th2 + Th3)*cos(Th4)*cos(Th5)) - 0.01294*sin(Th2 + Th3)*cos(Th5) - 0.01294*cos(Th2 + Th3)*cos(Th4)*sin(Th5) + 0.00023*cos(Th2 + Th3)*sin(Th4)*sin(Th6)))*(0.05206*cos(Th1)*cos(Th4)*sin(Th5) + 0.00023*cos(Th1)*sin(Th4)*sin(Th6) + 0.00023*sin(Th2 + Th3)*cos(Th4)*sin(Th1)*sin(Th6) - 0.05206*sin(Th2 + Th3)*sin(Th1)*sin(Th4)*sin(Th5) - 0.00023*cos(Th1)*cos(Th4)*cos(Th5)*cos(Th6) + 0.00023*sin(Th2 + Th3)*cos(Th5)*cos(Th6)*sin(Th1)*sin(Th4)) - (sin(Th2 + Th3)*cos(Th5) + cos(Th2 + Th3)*cos(Th4)*sin(Th5))*(cos(Th2 + Th3)*sin(Th1)*((0.00104*cos(Th6)*(cos(Th1)*cos(Th4) - 1.0*sin(Th2 + Th3)*sin(Th1)*sin(Th4)) - 0.00104*sin(Th6)*(cos(Th5)*(cos(Th1)*sin(Th4) + sin(Th2 + Th3)*cos(Th4)*sin(Th1)) + cos(Th2 + Th3)*sin(Th1)*sin(Th5)))*(sin(Th6)*(sin(Th2 + Th3)*sin(Th5) - 1.0*cos(Th2 + Th3)*cos(Th4)*cos(Th5)) - 1.0*cos(Th2 + Th3)*cos(Th6)*sin(Th4)) - (cos(Th6)*(sin(Th2 + Th3)*sin(Th5) - 1.0*cos(Th2 + Th3)*cos(Th4)*cos(Th5)) + cos(Th2 + Th3)*sin(Th4)*sin(Th6))*(0.001043*sin(Th6)*(cos(Th1)*cos(Th4) - 1.0*sin(Th2 + Th3)*sin(Th1)*sin(Th4)) + 0.001043*cos(Th6)*(cos(Th5)*(cos(Th1)*sin(Th4) + sin(Th2 + Th3)*cos(Th4)*sin(Th1)) + cos(Th2 + Th3)*sin(Th1)*sin(Th5)) + 4.0e-6*sin(Th5)*(cos(Th1)*sin(Th4) + sin(Th2 + Th3)*cos(Th4)*sin(Th1)) - 4.0e-6*cos(Th2 + Th3)*cos(Th5)*sin(Th1)) + 1.0*(sin(Th2 + Th3)*cos(Th5) + cos(Th2 + Th3)*cos(Th4)*sin(Th5))*(4.0e-6*sin(Th6)*(cos(Th1)*cos(Th4) - 1.0*sin(Th2 + Th3)*sin(Th1)*sin(Th4)) + 4.0e-6*cos(Th6)*(cos(Th5)*(cos(Th1)*sin(Th4) + sin(Th2 + Th3)*cos(Th4)*sin(Th1)) + cos(Th2 + Th3)*sin(Th1)*sin(Th5)) + 0.000116*sin(Th5)*(cos(Th1)*sin(Th4) + sin(Th2 + Th3)*cos(Th4)*sin(Th1)) - 0.000116*cos(Th2 + Th3)*cos(Th5)*sin(Th1))) - sin(Th2 + Th3)*((sin(Th6)*(sin(Th2 + Th3)*sin(Th5) - 1.0*cos(Th2 + Th3)*cos(Th4)*cos(Th5)) - 1.0*cos(Th2 + Th3)*cos(Th6)*sin(Th4))*(0.00104*sin(Th6)*(sin(Th2 + Th3)*sin(Th5) - 1.0*cos(Th2 + Th3)*cos(Th4)*cos(Th5)) - 0.00104*cos(Th2 + Th3)*cos(Th6)*sin(Th4)) - 1.0*(sin(Th2 + Th3)*cos(Th5) + cos(Th2 + Th3)*cos(Th4)*sin(Th5))*(4.0e-6*cos(Th6)*(sin(Th2 + Th3)*sin(Th5) - 1.0*cos(Th2 + Th3)*cos(Th4)*cos(Th5)) - 0.000116*sin(Th2 + Th3)*cos(Th5) - 0.000116*cos(Th2 + Th3)*cos(Th4)*sin(Th5) + 4.0e-6*cos(Th2 + Th3)*sin(Th4)*sin(Th6)) + (cos(Th6)*(sin(Th2 + Th3)*sin(Th5) - 1.0*cos(Th2 + Th3)*cos(Th4)*cos(Th5)) + cos(Th2 + Th3)*sin(Th4)*sin(Th6))*(0.001043*cos(Th6)*(sin(Th2 + Th3)*sin(Th5) - 1.0*cos(Th2 + Th3)*cos(Th4)*cos(Th5)) - 4.0e-6*sin(Th2 + Th3)*cos(Th5) - 4.0e-6*cos(Th2 + Th3)*cos(Th4)*sin(Th5) + 0.001043*cos(Th2 + Th3)*sin(Th4)*sin(Th6))) + 1.0*cos(Th2 + Th3)*cos(Th1)*((0.00104*sin(Th6)*(cos(Th5)*(sin(Th1)*sin(Th4) - 1.0*sin(Th2 + Th3)*cos(Th1)*cos(Th4)) - 1.0*cos(Th2 + Th3)*cos(Th1)*sin(Th5)) - 0.00104*cos(Th6)*(cos(Th4)*sin(Th1) + sin(Th2 + Th3)*cos(Th1)*sin(Th4)))*(sin(Th6)*(sin(Th2 + Th3)*sin(Th5) - 1.0*cos(Th2 + Th3)*cos(Th4)*cos(Th5)) - 1.0*cos(Th2 + Th3)*cos(Th6)*sin(Th4)) + (cos(Th6)*(sin(Th2 + Th3)*sin(Th5) - 1.0*cos(Th2 + Th3)*cos(Th4)*cos(Th5)) + cos(Th2 + Th3)*sin(Th4)*sin(Th6))*(4.0e-6*sin(Th5)*(sin(Th1)*sin(Th4) - 1.0*sin(Th2 + Th3)*cos(Th1)*cos(Th4)) + 0.001043*sin(Th6)*(cos(Th4)*sin(Th1) + sin(Th2 + Th3)*cos(Th1)*sin(Th4)) + 0.001043*cos(Th6)*(cos(Th5)*(sin(Th1)*sin(Th4) - 1.0*sin(Th2 + Th3)*cos(Th1)*cos(Th4)) - 1.0*cos(Th2 + Th3)*cos(Th1)*sin(Th5)) + 4.0e-6*cos(Th2 + Th3)*cos(Th1)*cos(Th5)) - 1.0*(sin(Th2 + Th3)*cos(Th5) + cos(Th2 + Th3)*cos(Th4)*sin(Th5))*(0.000116*sin(Th5)*(sin(Th1)*sin(Th4) - 1.0*sin(Th2 + Th3)*cos(Th1)*cos(Th4)) + 4.0e-6*sin(Th6)*(cos(Th4)*sin(Th1) + sin(Th2 + Th3)*cos(Th1)*sin(Th4)) + 4.0e-6*cos(Th6)*(cos(Th5)*(sin(Th1)*sin(Th4) - 1.0*sin(Th2 + Th3)*cos(Th1)*cos(Th4)) - 1.0*cos(Th2 + Th3)*cos(Th1)*sin(Th5)) + 0.000116*cos(Th2 + Th3)*cos(Th1)*cos(Th5)))) - 1.0*(0.5*(sin(Th5)*(cos(Th1)*sin(Th4) + sin(Th2 + Th3)*cos(Th4)*sin(Th1)) - 1.0*cos(Th2 + Th3)*cos(Th5)*sin(Th1))*(0.00023*cos(Th6)*(sin(Th2 + Th3)*sin(Th5) - 1.0*cos(Th2 + Th3)*cos(Th4)*cos(Th5)) - 0.01294*sin(Th2 + Th3)*cos(Th5) - 0.01294*cos(Th2 + Th3)*cos(Th4)*sin(Th5) + 0.00023*cos(Th2 + Th3)*sin(Th4)*sin(Th6)) + 0.5*(sin(Th2 + Th3)*cos(Th5) + cos(Th2 + Th3)*cos(Th4)*sin(Th5))*(0.00023*sin(Th6)*(cos(Th1)*cos(Th4) - 1.0*sin(Th2 + Th3)*sin(Th1)*sin(Th4)) + 0.00023*cos(Th6)*(cos(Th5)*(cos(Th1)*sin(Th4) + sin(Th2 + Th3)*cos(Th4)*sin(Th1)) + cos(Th2 + Th3)*sin(Th1)*sin(Th5)) + 0.01294*sin(Th5)*(cos(Th1)*sin(Th4) + sin(Th2 + Th3)*cos(Th4)*sin(Th1)) - 0.01294*cos(Th2 + Th3)*cos(Th5)*sin(Th1)))*(0.05206*cos(Th4)*sin(Th1)*sin(Th5) + 0.00023*sin(Th1)*sin(Th4)*sin(Th6) - 0.00023*sin(Th2 + Th3)*cos(Th1)*cos(Th4)*sin(Th6) + 0.05206*sin(Th2 + Th3)*cos(Th1)*sin(Th4)*sin(Th5) - 0.00023*cos(Th4)*cos(Th5)*cos(Th6)*sin(Th1) - 0.00023*sin(Th2 + Th3)*cos(Th1)*cos(Th5)*cos(Th6)*sin(Th4)) - 1.0*(sin(Th5)*(sin(Th1)*sin(Th4) - 1.0*sin(Th2 + Th3)*cos(Th1)*cos(Th4)) + cos(Th2 + Th3)*cos(Th1)*cos(Th5))*(sin(Th2 + Th3)*((0.00104*sin(Th6)*(sin(Th2 + Th3)*sin(Th5) - 1.0*cos(Th2 + Th3)*cos(Th4)*cos(Th5)) - 0.00104*cos(Th2 + Th3)*cos(Th6)*sin(Th4))*(sin(Th6)*(cos(Th5)*(sin(Th1)*sin(Th4) - 1.0*sin(Th2 + Th3)*cos(Th1)*cos(Th4)) - 1.0*cos(Th2 + Th3)*cos(Th1)*sin(Th5)) - 1.0*cos(Th6)*(cos(Th4)*sin(Th1) + sin(Th2 + Th3)*cos(Th1)*sin(Th4))) + (sin(Th6)*(cos(Th4)*sin(Th1) + sin(Th2 + Th3)*cos(Th1)*sin(Th4)) + cos(Th6)*(cos(Th5)*(sin(Th1)*sin(Th4) - 1.0*sin(Th2 + Th3)*cos(Th1)*cos(Th4)) - 1.0*cos(Th2 + Th3)*cos(Th1)*sin(Th5)))*(0.001043*cos(Th6)*(sin(Th2 + Th3)*sin(Th5) - 1.0*cos(Th2 + Th3)*cos(Th4)*cos(Th5)) - 4.0e-6*sin(Th2 + Th3)*cos(Th5) - 4.0e-6*cos(Th2 + Th3)*cos(Th4)*sin(Th5) + 0.001043*cos(Th2 + Th3)*sin(Th4)*sin(Th6)) + (sin(Th5)*(sin(Th1)*sin(Th4) - 1.0*sin(Th2 + Th3)*cos(Th1)*cos(Th4)) + cos(Th2 + Th3)*cos(Th1)*cos(Th5))*(4.0e-6*cos(Th6)*(sin(Th2 + Th3)*sin(Th5) - 1.0*cos(Th2 + Th3)*cos(Th4)*cos(Th5)) - 0.000116*sin(Th2 + Th3)*cos(Th5) - 0.000116*cos(Th2 + Th3)*cos(Th4)*sin(Th5) + 4.0e-6*cos(Th2 + Th3)*sin(Th4)*sin(Th6))) - 1.0*cos(Th2 + Th3)*cos(Th1)*((0.00104*sin(Th6)*(cos(Th5)*(sin(Th1)*sin(Th4) - 1.0*sin(Th2 + Th3)*cos(Th1)*cos(Th4)) - 1.0*cos(Th2 + Th3)*cos(Th1)*sin(Th5)) - 0.00104*cos(Th6)*(cos(Th4)*sin(Th1) + sin(Th2 + Th3)*cos(Th1)*sin(Th4)))*(sin(Th6)*(cos(Th5)*(sin(Th1)*sin(Th4) - 1.0*sin(Th2 + Th3)*cos(Th1)*cos(Th4)) - 1.0*cos(Th2 + Th3)*cos(Th1)*sin(Th5)) - 1.0*cos(Th6)*(cos(Th4)*sin(Th1) + sin(Th2 + Th3)*cos(Th1)*sin(Th4))) + (sin(Th6)*(cos(Th4)*sin(Th1) + sin(Th2 + Th3)*cos(Th1)*sin(Th4)) + cos(Th6)*(cos(Th5)*(sin(Th1)*sin(Th4) - 1.0*sin(Th2 + Th3)*cos(Th1)*cos(Th4)) - 1.0*cos(Th2 + Th3)*cos(Th1)*sin(Th5)))*(4.0e-6*sin(Th5)*(sin(Th1)*sin(Th4) - 1.0*sin(Th2 + Th3)*cos(Th1)*cos(Th4)) + 0.001043*sin(Th6)*(cos(Th4)*sin(Th1) + sin(Th2 + Th3)*cos(Th1)*sin(Th4)) + 0.001043*cos(Th6)*(cos(Th5)*(sin(Th1)*sin(Th4) - 1.0*sin(Th2 + Th3)*cos(Th1)*cos(Th4)) - 1.0*cos(Th2 + Th3)*cos(Th1)*sin(Th5)) + 4.0e-6*cos(Th2 + Th3)*cos(Th1)*cos(Th5)) + (sin(Th5)*(sin(Th1)*sin(Th4) - 1.0*sin(Th2 + Th3)*cos(Th1)*cos(Th4)) + cos(Th2 + Th3)*cos(Th1)*cos(Th5))*(0.000116*sin(Th5)*(sin(Th1)*sin(Th4) - 1.0*sin(Th2 + Th3)*cos(Th1)*cos(Th4)) + 4.0e-6*sin(Th6)*(cos(Th4)*sin(Th1) + sin(Th2 + Th3)*cos(Th1)*sin(Th4)) + 4.0e-6*cos(Th6)*(cos(Th5)*(sin(Th1)*sin(Th4) - 1.0*sin(Th2 + Th3)*cos(Th1)*cos(Th4)) - 1.0*cos(Th2 + Th3)*cos(Th1)*sin(Th5)) + 0.000116*cos(Th2 + Th3)*cos(Th1)*cos(Th5))) + cos(Th2 + Th3)*sin(Th1)*((sin(Th6)*(cos(Th4)*sin(Th1) + sin(Th2 + Th3)*cos(Th1)*sin(Th4)) + cos(Th6)*(cos(Th5)*(sin(Th1)*sin(Th4) - 1.0*sin(Th2 + Th3)*cos(Th1)*cos(Th4)) - 1.0*cos(Th2 + Th3)*cos(Th1)*sin(Th5)))*(0.001043*sin(Th6)*(cos(Th1)*cos(Th4) - 1.0*sin(Th2 + Th3)*sin(Th1)*sin(Th4)) + 0.001043*cos(Th6)*(cos(Th5)*(cos(Th1)*sin(Th4) + sin(Th2 + Th3)*cos(Th4)*sin(Th1)) + cos(Th2 + Th3)*sin(Th1)*sin(Th5)) + 4.0e-6*sin(Th5)*(cos(Th1)*sin(Th4) + sin(Th2 + Th3)*cos(Th4)*sin(Th1)) - 4.0e-6*cos(Th2 + Th3)*cos(Th5)*sin(Th1)) + (sin(Th5)*(sin(Th1)*sin(Th4) - 1.0*sin(Th2 + Th3)*cos(Th1)*cos(Th4)) + cos(Th2 + Th3)*cos(Th1)*cos(Th5))*(4.0e-6*sin(Th6)*(cos(Th1)*cos(Th4) - 1.0*sin(Th2 + Th3)*sin(Th1)*sin(Th4)) + 4.0e-6*cos(Th6)*(cos(Th5)*(cos(Th1)*sin(Th4) + sin(Th2 + Th3)*cos(Th4)*sin(Th1)) + cos(Th2 + Th3)*sin(Th1)*sin(Th5)) + 0.000116*sin(Th5)*(cos(Th1)*sin(Th4) + sin(Th2 + Th3)*cos(Th4)*sin(Th1)) - 0.000116*cos(Th2 + Th3)*cos(Th5)*sin(Th1)) - (0.00104*cos(Th6)*(cos(Th1)*cos(Th4) - 1.0*sin(Th2 + Th3)*sin(Th1)*sin(Th4)) - 0.00104*sin(Th6)*(cos(Th5)*(cos(Th1)*sin(Th4) + sin(Th2 + Th3)*cos(Th4)*sin(Th1)) + cos(Th2 + Th3)*sin(Th1)*sin(Th5)))*(sin(Th6)*(cos(Th5)*(sin(Th1)*sin(Th4) - 1.0*sin(Th2 + Th3)*cos(Th1)*cos(Th4)) - 1.0*cos(Th2 + Th3)*cos(Th1)*sin(Th5)) - 1.0*cos(Th6)*(cos(Th4)*sin(Th1) + sin(Th2 + Th3)*cos(Th1)*sin(Th4))))) - 1.0*(sin(Th5)*(cos(Th1)*sin(Th4) + sin(Th2 + Th3)*cos(Th4)*sin(Th1)) - 1.0*cos(Th2 + Th3)*cos(Th5)*sin(Th1))*(sin(Th2 + Th3)*((sin(Th6)*(cos(Th1)*cos(Th4) - 1.0*sin(Th2 + Th3)*sin(Th1)*sin(Th4)) + cos(Th6)*(cos(Th5)*(cos(Th1)*sin(Th4) + sin(Th2 + Th3)*cos(Th4)*sin(Th1)) + cos(Th2 + Th3)*sin(Th1)*sin(Th5)))*(0.001043*cos(Th6)*(sin(Th2 + Th3)*sin(Th5) - 1.0*cos(Th2 + Th3)*cos(Th4)*cos(Th5)) - 4.0e-6*sin(Th2 + Th3)*cos(Th5) - 4.0e-6*cos(Th2 + Th3)*cos(Th4)*sin(Th5) + 0.001043*cos(Th2 + Th3)*sin(Th4)*sin(Th6)) + (sin(Th5)*(cos(Th1)*sin(Th4) + sin(Th2 + Th3)*cos(Th4)*sin(Th1)) - 1.0*cos(Th2 + Th3)*cos(Th5)*sin(Th1))*(4.0e-6*cos(Th6)*(sin(Th2 + Th3)*sin(Th5) - 1.0*cos(Th2 + Th3)*cos(Th4)*cos(Th5)) - 0.000116*sin(Th2 + Th3)*cos(Th5) - 0.000116*cos(Th2 + Th3)*cos(Th4)*sin(Th5) + 4.0e-6*cos(Th2 + Th3)*sin(Th4)*sin(Th6)) - (1.0*cos(Th6)*(cos(Th1)*cos(Th4) - 1.0*sin(Th2 + Th3)*sin(Th1)*sin(Th4)) - sin(Th6)*(cos(Th5)*(cos(Th1)*sin(Th4) + sin(Th2 + Th3)*cos(Th4)*sin(Th1)) + cos(Th2 + Th3)*sin(Th1)*sin(Th5)))*(0.00104*sin(Th6)*(sin(Th2 + Th3)*sin(Th5) - 1.0*cos(Th2 + Th3)*cos(Th4)*cos(Th5)) - 0.00104*cos(Th2 + Th3)*cos(Th6)*sin(Th4))) - 1.0*cos(Th2 + Th3)*cos(Th1)*((sin(Th6)*(cos(Th1)*cos(Th4) - 1.0*sin(Th2 + Th3)*sin(Th1)*sin(Th4)) + cos(Th6)*(cos(Th5)*(cos(Th1)*sin(Th4) + sin(Th2 + Th3)*cos(Th4)*sin(Th1)) + cos(Th2 + Th3)*sin(Th1)*sin(Th5)))*(4.0e-6*sin(Th5)*(sin(Th1)*sin(Th4) - 1.0*sin(Th2 + Th3)*cos(Th1)*cos(Th4)) + 0.001043*sin(Th6)*(cos(Th4)*sin(Th1) + sin(Th2 + Th3)*cos(Th1)*sin(Th4)) + 0.001043*cos(Th6)*(cos(Th5)*(sin(Th1)*sin(Th4) - 1.0*sin(Th2 + Th3)*cos(Th1)*cos(Th4)) - 1.0*cos(Th2 + Th3)*cos(Th1)*sin(Th5)) + 4.0e-6*cos(Th2 + Th3)*cos(Th1)*cos(Th5)) - (0.00104*sin(Th6)*(cos(Th5)*(sin(Th1)*sin(Th4) - 1.0*sin(Th2 + Th3)*cos(Th1)*cos(Th4)) - 1.0*cos(Th2 + Th3)*cos(Th1)*sin(Th5)) - 0.00104*cos(Th6)*(cos(Th4)*sin(Th1) + sin(Th2 + Th3)*cos(Th1)*sin(Th4)))*(1.0*cos(Th6)*(cos(Th1)*cos(Th4) - 1.0*sin(Th2 + Th3)*sin(Th1)*sin(Th4)) - sin(Th6)*(cos(Th5)*(cos(Th1)*sin(Th4) + sin(Th2 + Th3)*cos(Th4)*sin(Th1)) + cos(Th2 + Th3)*sin(Th1)*sin(Th5))) + (sin(Th5)*(cos(Th1)*sin(Th4) + sin(Th2 + Th3)*cos(Th4)*sin(Th1)) - 1.0*cos(Th2 + Th3)*cos(Th5)*sin(Th1))*(0.000116*sin(Th5)*(sin(Th1)*sin(Th4) - 1.0*sin(Th2 + Th3)*cos(Th1)*cos(Th4)) + 4.0e-6*sin(Th6)*(cos(Th4)*sin(Th1) + sin(Th2 + Th3)*cos(Th1)*sin(Th4)) + 4.0e-6*cos(Th6)*(cos(Th5)*(sin(Th1)*sin(Th4) - 1.0*sin(Th2 + Th3)*cos(Th1)*cos(Th4)) - 1.0*cos(Th2 + Th3)*cos(Th1)*sin(Th5)) + 0.000116*cos(Th2 + Th3)*cos(Th1)*cos(Th5))) + cos(Th2 + Th3)*sin(Th1)*((0.00104*cos(Th6)*(cos(Th1)*cos(Th4) - 1.0*sin(Th2 + Th3)*sin(Th1)*sin(Th4)) - 0.00104*sin(Th6)*(cos(Th5)*(cos(Th1)*sin(Th4) + sin(Th2 + Th3)*cos(Th4)*sin(Th1)) + cos(Th2 + Th3)*sin(Th1)*sin(Th5)))*(1.0*cos(Th6)*(cos(Th1)*cos(Th4) - 1.0*sin(Th2 + Th3)*sin(Th1)*sin(Th4)) - sin(Th6)*(cos(Th5)*(cos(Th1)*sin(Th4) + sin(Th2 + Th3)*cos(Th4)*sin(Th1)) + cos(Th2 + Th3)*sin(Th1)*sin(Th5))) + (sin(Th5)*(cos(Th1)*sin(Th4) + sin(Th2 + Th3)*cos(Th4)*sin(Th1)) - 1.0*cos(Th2 + Th3)*cos(Th5)*sin(Th1))*(4.0e-6*sin(Th6)*(cos(Th1)*cos(Th4) - 1.0*sin(Th2 + Th3)*sin(Th1)*sin(Th4)) + 4.0e-6*cos(Th6)*(cos(Th5)*(cos(Th1)*sin(Th4) + sin(Th2 + Th3)*cos(Th4)*sin(Th1)) + cos(Th2 + Th3)*sin(Th1)*sin(Th5)) + 0.000116*sin(Th5)*(cos(Th1)*sin(Th4) + sin(Th2 + Th3)*cos(Th4)*sin(Th1)) - 0.000116*cos(Th2 + Th3)*cos(Th5)*sin(Th1)) + (sin(Th6)*(cos(Th1)*cos(Th4) - 1.0*sin(Th2 + Th3)*sin(Th1)*sin(Th4)) + cos(Th6)*(cos(Th5)*(cos(Th1)*sin(Th4) + sin(Th2 + Th3)*cos(Th4)*sin(Th1)) + cos(Th2 + Th3)*sin(Th1)*sin(Th5)))*(0.001043*sin(Th6)*(cos(Th1)*cos(Th4) - 1.0*sin(Th2 + Th3)*sin(Th1)*sin(Th4)) + 0.001043*cos(Th6)*(cos(Th5)*(cos(Th1)*sin(Th4) + sin(Th2 + Th3)*cos(Th4)*sin(Th1)) + cos(Th2 + Th3)*sin(Th1)*sin(Th5)) + 4.0e-6*sin(Th5)*(cos(Th1)*sin(Th4) + sin(Th2 + Th3)*cos(Th4)*sin(Th1)) - 4.0e-6*cos(Th2 + Th3)*cos(Th5)*sin(Th1)))) + 0.5*cos(Th2 + Th3)*(0.00023*cos(Th4)*sin(Th6) - 0.05206*sin(Th4)*sin(Th5) + 0.00023*cos(Th5)*cos(Th6)*sin(Th4))*(0.00023*cos(Th2 + Th3)*cos(Th6)*sin(Th4) - 0.00023*sin(Th2 + Th3)*sin(Th5)*sin(Th6) + 0.00023*cos(Th2 + Th3)*cos(Th4)*cos(Th5)*sin(Th6));
% M61=M16; M31=M13; M41=M14; M51=M15; M21=M12;
end
